simulink model "lab1"  (R2021a)
settings: Solver=VariableStepAuto  StartTime=0.0  StopTime=30  RelTol=1e-3
undefined symbols (not defined in the file): b1, b2, b3, F_1, F_2, j1, j2, k1, k2, k3, time_F_1, time_F_2, x1_0, x2_0
settings Model: Creator=Alex  LastModifiedBy=Alex

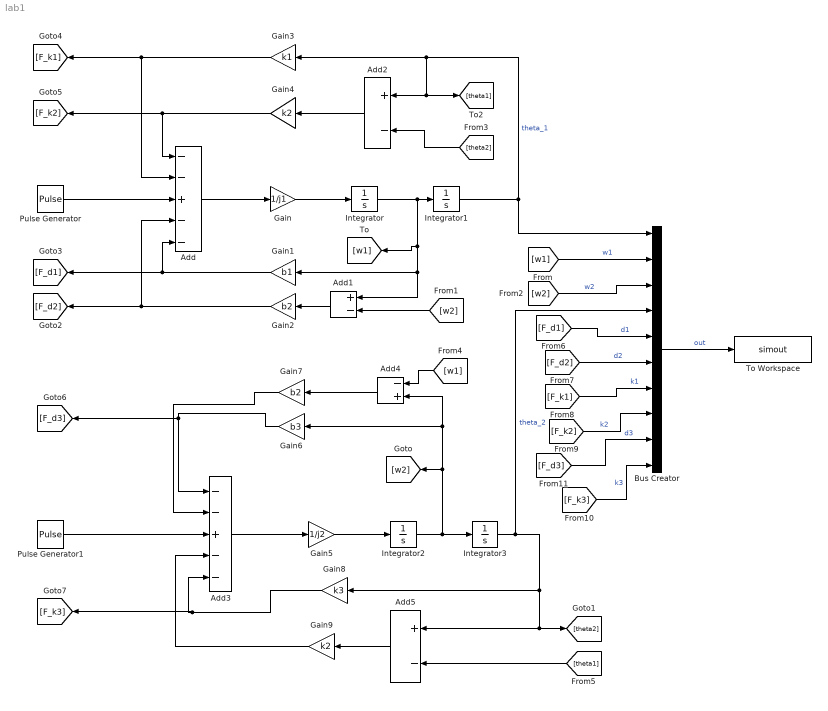
== system lab1 ==
  Add : Sum  Inputs=--+--
  Add1 : Sum  Inputs=+-
  Add2 : Sum  Inputs=+-
  Add3 : Sum  Inputs=--+--
  Add4 : Sum  Inputs=-+
  Add5 : Sum  Inputs=+-
  Bus Creator : BusCreator  Inputs=10
  Gain : Gain  Gain=1/j1
  Gain1 : Gain  Gain=b1
  Gain2 : Gain  Gain=b2
  Gain3 : Gain  Gain=k1
  Gain4 : Gain  Gain=k2
  Gain5 : Gain  Gain=1/j2
  Gain6 : Gain  Gain=b3
  Gain7 : Gain  Gain=b2
  Gain8 : Gain  Gain=k3
  Gain9 : Gain  Gain=k2
  Integrator : Integrator
  Integrator1 : Integrator  InitialCondition=x1_0
  Integrator2 : Integrator
  Integrator3 : Integrator  InitialCondition=x2_0
  Pulse Generator : DiscretePulseGenerator  PulseType=Time based  Amplitude=F_1  Period=t+10  PulseWidth=100 * time_F_1 / (t + 10)
  Pulse Generator1 : DiscretePulseGenerator  PulseType=Time based  Amplitude=F_2  Period=t+10  PulseWidth=100 * time_F_2 / (t + 10)
  To Workspace : ToWorkspace  VariableName=simout  SaveFormat=Timeseries  SampleTime=-1
  wires:
  Gain/1 -> Integrator/1
  [w1] -> Bus Creator/2  "w1"
  Add/1 -> Gain/1
  Gain1/1 -> [F_d1], Add/5
  Gain2/1 -> [F_d2], Add/4
  Integrator/1 -> Add1/1, Gain1/1, [w1], Integrator1/1
  Add1/1 -> Gain2/1
  [w2] -> Add1/2
  Gain3/1 -> [F_k1], Add/2
  Gain4/1 -> [F_k2], Add/1
  Integrator1/1 -> [theta1], Add2/1, Gain3/1, Bus Creator/1  "theta_1"
  Add2/1 -> Gain4/1
  [theta2] -> Add2/2
  Gain5/1 -> Integrator2/1
  Integrator2/1 -> Add4/2, Gain6/1, [w2], Integrator3/1
  [w2] -> Bus Creator/3  "w2"
  Bus Creator/1 -> To Workspace/1  "out"
  Add3/1 -> Gain5/1
  Integrator3/1 -> Gain8/1, Add5/1, [theta2], Bus Creator/4  "theta_2"
  Gain6/1 -> [F_d3], Add3/1
  [w1] -> Add4/1
  Add4/1 -> Gain7/1
  Gain7/1 -> Add3/2
  Add5/1 -> Gain9/1
  [theta1] -> Add5/2
  Pulse Generator/1 -> Add/3
  Gain9/1 -> Add3/4
  Gain8/1 -> [F_k3], Add3/5
  Pulse Generator1/1 -> Add3/3
  [F_d1] -> Bus Creator/5  "d1"
  [F_d2] -> Bus Creator/6  "d2"
  [F_k1] -> Bus Creator/7  "k1"
  [F_k2] -> Bus Creator/8  "k2"
  [F_k3] -> Bus Creator/10  "k3"
  [F_d3] -> Bus Creator/9  "d3"
